simulink model "simulink_test_bt_lvp"  (R2024a)
settings: Solver=VariableStepAuto  StartTime=0.0  StopTime=10.0  RelTol=1e-1
values from neighbouring files (symbols this model uses):
  r1 = BodyTree(J1, B1)    [test_simulink_lvp.m]
libraries: SoftRobotics x1
settings Model: Creator=pietro  LastModifiedBy=pietro
settings SolverCC: ShapePreserveControl=EnableAll  ZeroCrossAlgorithm=Adaptive  SolverResetMethod=Robust
settings RTWCC: GenerateReport=on  GPUComputeCapability=3.5

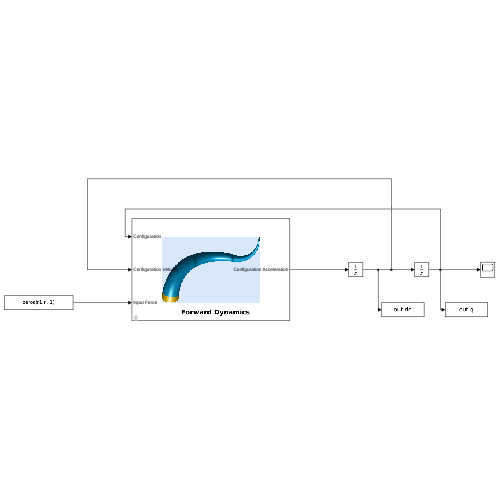
[thumbnail: Simulink's stored preview of the top-level diagram]
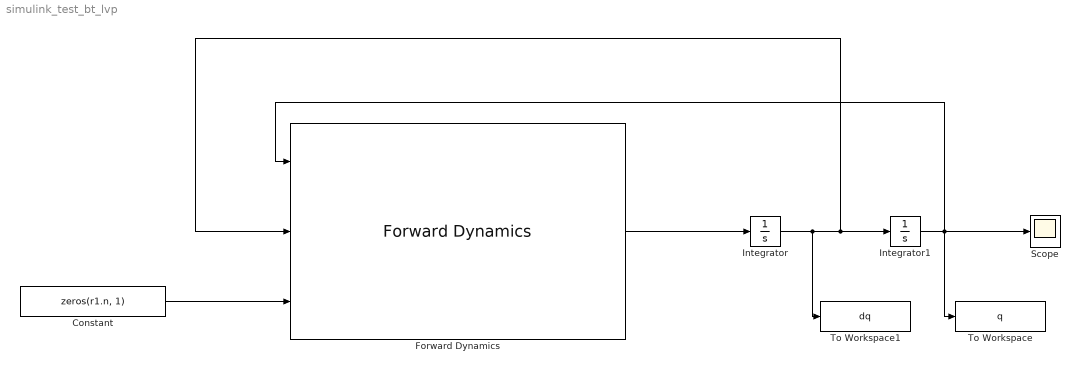
== system simulink_test_bt_lvp ==
  Constant : Constant  Value=zeros(r1.n, 1)
  Forward Dynamics : SoftRobotics/Forward Dynamics  RobotModel=r1  SimulateUsing=Code generation
      settings: SourceProductName=Jelly
  Integrator : Integrator
  Integrator1 : Integrator  InitialCondition=zeros(r1.n, 1)
  Scope : Scope
  To Workspace : ToWorkspace  VariableName=q  SaveFormat=Timeseries  SampleTime=-1
  To Workspace1 : ToWorkspace  VariableName=dq  SaveFormat=Timeseries  SampleTime=-1
  wires:
  Forward Dynamics/1 -> Integrator/1
  Integrator/1 -> To Workspace1/1, Forward Dynamics/2, Integrator1/1
  Constant/1 -> Forward Dynamics/3
  Integrator1/1 -> To Workspace/1, Forward Dynamics/1, Scope/1
